simulink model "posture_regulation"  (R2025b)
settings: Solver=VariableStepAuto  StartTime=0.0  StopTime=30  RelTol=1e-3
libraries: robotmobilelib x1
settings Model: Creator=alessandrochinello  LastModifiedBy=luca

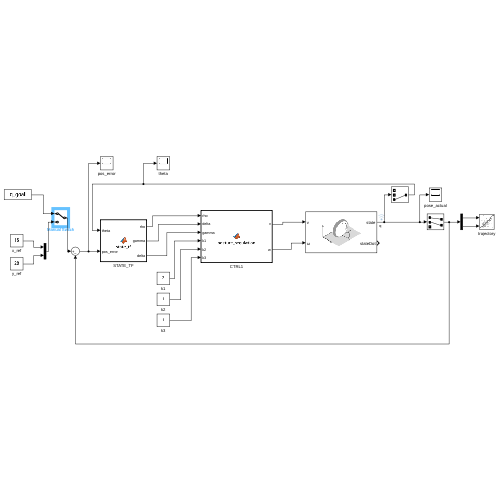
[thumbnail: Simulink's stored preview of the top-level diagram]
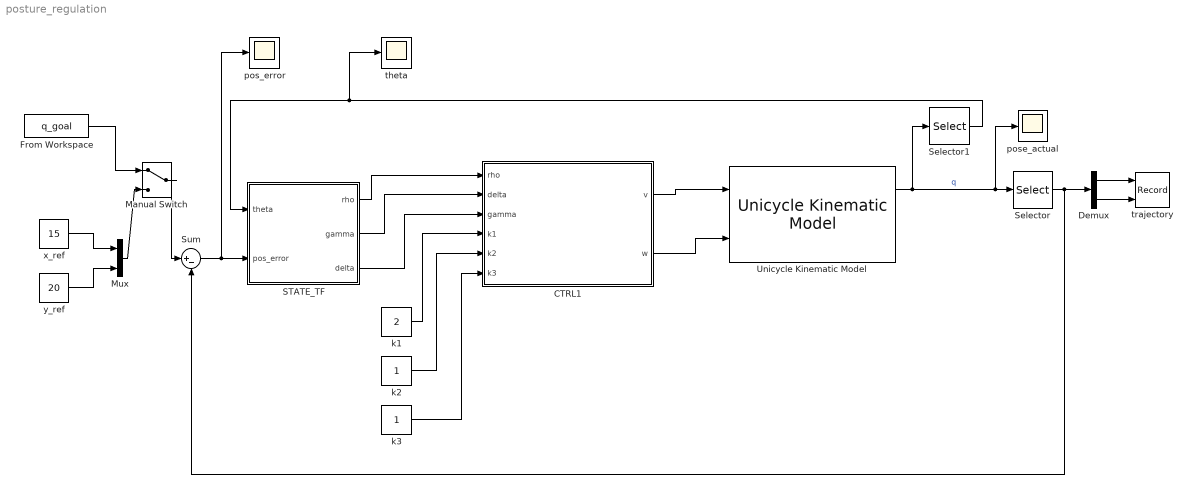
== system posture_regulation ==
  CTRL1 : MATLAB Function  TreatAsAtomicUnit=on
  Demux : Demux  Outputs=2
  From Workspace : FromWorkspace  VariableName=q_goal
  Manual Switch : ManualSwitch
  Mux : Mux  Inputs=2
  STATE_TF : MATLAB Function  TreatAsAtomicUnit=on
  Selector : Selector  InputPortWidth=3  IndexOptions=Index vector (dialog)  Indices=[1 2]  OutputSizes=1
  Selector1 : Selector  InputPortWidth=3  IndexOptions=Index vector (dialog)  Indices=[3]  OutputSizes=1
  Sum : Sum  Inputs=|+-
  Unicycle Kinematic Model : robotmobilelib/Unicycle Kinematic Model  VehicleInputs=Vehicle Speed & Heading Angular Velocity  WheelRadius=0.1  WheelSpeedRange=[-Inf Inf]  InitialState=[0; 0; 0]  SimulateUsing=Interpreted execution
  k1 : Constant  Value=2
  k2 : Constant
  k3 : Constant
  pos_error : Scope
      settings: ActiveDisplayYMinimum=-418.45288489633356  ActiveDisplayYMaximum=248.82865119862322
  pose_actual : Scope
      settings: ActiveDisplayYMinimum=-37.155041353571882  ActiveDisplayYMaximum=8.5892802665132866
  theta : Scope
      settings: ActiveDisplayYMinimum=-1826.061877140877  ActiveDisplayYMaximum=1403.1503315532193  DataLoggingVariableName=ScopeData2
  trajectory : Record  NumPorts=2.0  FileSettingsInternal="{\"entries\":[{\"content\":{\"excelSettings\":{\"content\":{},\"type\":\"Streamout.ExcelSettings\"},\"parquetSettings\":{\"content\":{},\"type\":\"Streamout.ParquetSettings\"}},\"type\":\"Streamout.FileSettingStorage\",\"uuid\":\"\"}],\"packageUris\":[\"http:\\/\\/schema.mathworks.com\\/mf0\\/streamout_blocks\\/R2020a\"],\"version\":\"1.0\"}"  FrameSettings=[0, 0]  Layout=[1 1]  SignalsInternal="{\"entries\":[{\"content\":{\"signals\":[{\"content\":{\"blockPath\":[],\"dimensions\":[1],\"domain\":\"\",\"lineColor\":\"#a2142f\",\"plots\":[ 1 ],\"port\":1,\"sid\":[\"\"],\"signalID\":1,\"signalName\":\"Demux:1\"},\"type\":\"RecordBlkView.Signal\",\"uuid\":\"\"},{\"content\":{\"blockPath\":[],\"dimensions\":[1],\"domain\":\"\",\"lineColor\":\"#139fff\",\"plots\":[ 1 ],\"port\":2,\"sid\":[\"\"],\"signalID\":2,\"signalName\":\"Demux:2\"},\"type\":\"RecordBlkView.Signal\",\"uuid\":\"\"}]},\"type\":\"RecordBlkView.InputSignals\",\"uuid\":\"\"}],\"packageUris\":[\"http:\\/\\/schema.mathworks.com\\/mf0\\/streamout_blocks\\/R2020a\"],\"version\":\"1.0\"}"  VisualizationBindings="{\"xyplotplugin\":{\"info\":[{\"series\":[{\"bindingParametersList\":[{\"parameter\":\"X-Axis\",\"signalID\":1,\"signalName\":\"Demux:1\"},{\"parameter\":\"Y-Axis\",\"signalID\":2,\"signalName\":\"Demux:2\"}],\"seriesID\":0}],\"subplotID\":1}]}}"  CompatibilityTag=XY
  x_ref : Constant  Value=15
  y_ref : Constant  Value=20
  wires:
  x_ref/1 -> Mux/1
  y_ref/1 -> Mux/2
  Unicycle Kinematic Model/1 -> Selector1/1, pose_actual/1, Selector/1  "q"
  Demux/1 -> trajectory/1
  Demux/2 -> trajectory/2
  Selector/1 -> Demux/1, Sum/2
  From Workspace/1 -> Manual Switch/1
  Mux/1 -> Manual Switch/2
  Manual Switch/1 -> Sum/1
  Sum/1 -> pos_error/1, STATE_TF/2(pos_error)
  k1/1 -> CTRL1/4(k1)
  k2/1 -> CTRL1/5(k2)
  STATE_TF/1(rho) -> CTRL1/1(rho)
  STATE_TF/2(gamma) -> CTRL1/2(delta)
  STATE_TF/3(delta) -> CTRL1/3(gamma)
  CTRL1/2(w) -> Unicycle Kinematic Model/2
  CTRL1/1(v) -> Unicycle Kinematic Model/1
  Selector1/1 -> theta/1, STATE_TF/1(theta)
  k3/1 -> CTRL1/6(k3)

== matlab function posture_regulation/STATE_TF ==
  data: theta input; pos_error input; rho output; gamma output; delta output
function[rho, gamma, delta] = state_tf(theta, pos_error)

rho = sqrt(pos_error(1)^2 + pos_error(2)^2);

target_angle = atan2(pos_error(2), pos_error(1));
gamma = wrapToPi(target_angle - theta);

delta = wrapToPi(gamma + theta); %

end

== matlab function posture_regulation/CTRL1 ==
  data: rho input; delta input; gamma input; v output; w output; k1 input; k2 input; k3 input
function [v, w] = posture_regulation(rho, delta, gamma, k1, k2, k3)

u = k1 * cos(gamma);
v = rho * u;


if abs(gamma) < 1e-4
   sinc_val = 1;
else
   sinc_val = sin(gamma) * cos(gamma) / gamma;
end

w = k2 * gamma + k1 * sinc_val * (gamma + k3 * delta);

end
